simulink model "Modelo_Ceres_RetroROS"  (R2018b)
settings: Solver=VariableStepAuto  StartTime=0.0  StopTime=200  RelTol=1e-3
undefined symbols (not defined in the file): Angular, gainBruit, K_1, K_2, lim, Linear, Tao_1, Tao_2, X, Z
libraries: robotlib x5, simulink x4, realtime_pacer_lib x2
settings Model: Creator=adrir  LastModifiedBy=root
settings DebuggingCC: LibraryContextMissingDiagnostic=none
settings SFSimCC: SimUseLocalCustomCode=off
settings RTWCC: RTWUseLocalCustomCode=off
settings CodeAppCC: StateflowObjectComments=on

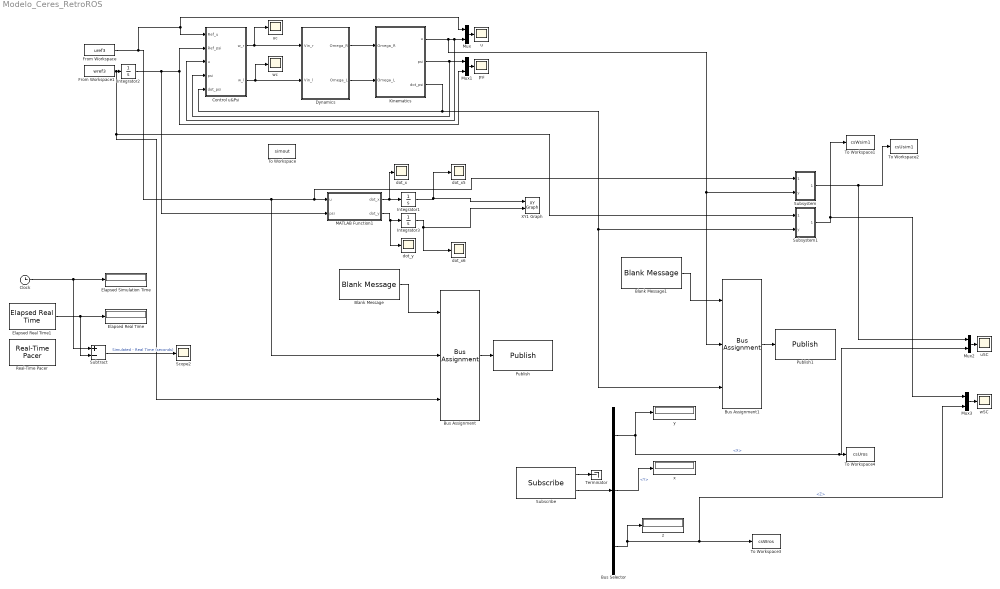
== system Modelo_Ceres_RetroROS ==
  Blank Message : robotlib/Blank Message  messageClass=Message  entityType=geometry_msgs/Twist  messageType=geometry_msgs/Twist  SampleTime=-1
      settings: SourceProductBaseCode=RO
  Blank Message1 : robotlib/Blank Message  messageClass=Message  entityType=geometry_msgs/Vector3  messageType=geometry_msgs/Vector3  SampleTime=-1
      settings: SourceProductBaseCode=RO
  Bus Assignment : BusAssignment  AssignedSignals=Linear.X,Angular.Z
  Bus Assignment1 : BusAssignment  AssignedSignals=X,Z
  Bus Selector : BusSelector  OutputSignals=X,Y,Z
  Clock : Clock
  Control u&Psi : Subsystem
  Dynamics : Subsystem
  Elapsed Real Time : Display
      settings: Decimation=2
  Elapsed Real Time1 : realtime_pacer_lib/Elapsed Real Time
  Elapsed Simulation Time : Display
      settings: Decimation=2
  From Workspace : FromWorkspace  VariableName=uref3
  From Workspace1 : FromWorkspace  VariableName=wref3
  Integrator1 : Integrator
  Integrator2 : Integrator
  Integrator3 : Integrator
  Kinematics : Subsystem
  MATLAB Function1 : MATLAB Function  TreatAsAtomicUnit=on
  Mux{,1..3} (4 alike) : Mux  Inputs=2
  Publish : robotlib/Publish  topicSource=Specify your own  topic=/ceres/cmd_vel  messageType=geometry_msgs/Twist  messageQueueLength=1
      settings: SourceProductBaseCode=RO
  Publish1 : robotlib/Publish  topicSource=Specify your own  topic=/advanced_navigation_driver/twist2D  messageType=geometry_msgs/Vector3  messageQueueLength=1
      settings: SourceProductBaseCode=RO
  Real-Time Pacer : realtime_pacer_lib/Real-Time Pacer  simTimePerRealTime=1
  Scope2 : Scope
  Subscribe : robotlib/Subscribe  topicSource=Select from ROS network  topic=/ceres/controlSignal  messageType=geometry_msgs/Vector3  sampleTime=-1  messageQueueLength=1
      settings: SourceProductBaseCode=RO
  Subsystem : Subsystem
  Subsystem1 : Subsystem
  Subtract : Sum  Inputs=+-
  Terminator : Terminator
  To Workspace : ToWorkspace  VariableName=simout  SaveFormat=Timeseries  SampleTime=-1
  To Workspace1 : ToWorkspace  VariableName=csWsim1  SaveFormat=Timeseries  SampleTime=-1
  To Workspace2 : ToWorkspace  VariableName=csUsim1  SaveFormat=Timeseries  SampleTime=-1
  To Workspace3 : ToWorkspace  VariableName=csWros  SaveFormat=Timeseries  SampleTime=-1
  To Workspace4 : ToWorkspace  VariableName=csUros  SaveFormat=Timeseries  SampleTime=-1
  XY1 Graph : simulink/Sinks/XY Graph  xmin=-30  xmax=30  ymin=-30  ymax=30  st=-1
  dot_x : Scope
  dot_x5 : Scope
  dot_x6 : Scope
  dot_y : Scope
  psi : Scope
  u : Scope
  uSC : Scope
  uc : Scope
  wSC : Scope
  wc : Scope
  x : Display
  y : Display
  z : Display
  wires:
  Dynamics/1(Omega_R) -> Kinematics/1(Omega_R)
  Dynamics/2(Omega_L) -> Kinematics/2(Omega_L)
  Kinematics/2(psi) -> Control u&Psi/4(psi), Mux1/1
  From Workspace/1 -> Control u&Psi/1(Ref_u), Mux/1, Bus Assignment/2, Subsystem/1(Ref), MATLAB Function1/1(u)
  Integrator2/1 -> Control u&Psi/2(Ref_psi), Mux1/2, MATLAB Function1/2(psi)
  Mux/1 -> u/1
  Mux1/1 -> psi/1
  Control u&Psi/1(w_r) -> uc/1, Dynamics/1(Vin_r)
  Control u&Psi/2(w_l) -> wc/1, Dynamics/2(Vin_l)
  Elapsed Real Time1/1 -> Elapsed Real Time/1, Subtract/2
  Subtract/1 -> Scope2/1  "Simulated - Real Time (seconds)"
  Integrator1/1 -> XY1 Graph/1, dot_x5/1
  Bus Assignment/1 -> Publish/1
  From Workspace1/1 -> Subsystem1/1(Ref), Bus Assignment/3, Integrator2/1
  MATLAB Function1/1(dot_x) -> dot_x/1, Integrator1/1
  Integrator3/1 -> XY1 Graph/2, dot_x6/1
  Blank Message/1 -> Bus Assignment/1
  MATLAB Function1/2(dot_y) -> dot_y/1, Integrator3/1
  Clock/1 -> Elapsed Simulation Time/1, Subtract/1
  Kinematics/1(u) -> Bus Assignment1/2, Subsystem/2(y), Control u&Psi/3(u), Mux/2
  Kinematics/3(dot_psi) -> Subsystem1/2(y), Bus Assignment1/3, Control u&Psi/5(dot_psi)
  Bus Assignment1/1 -> Publish1/1
  Blank Message1/1 -> Bus Assignment1/1
  Bus Selector/3 -> z/1, Mux3/2, To Workspace3/1  "<Z>"
  Subscribe/1 -> Terminator/1
  Subscribe/2 -> Bus Selector/1
  Bus Selector/2 -> x/1  "<Y>"
  Bus Selector/1 -> y/1, Mux2/2, To Workspace4/1  "<X>"
  Subsystem/1(c_u) -> Mux2/1, To Workspace2/1
  Subsystem1/1(c_psi) -> Mux3/1, To Workspace1/1
  Mux2/1 -> uSC/1
  Mux3/1 -> wSC/1

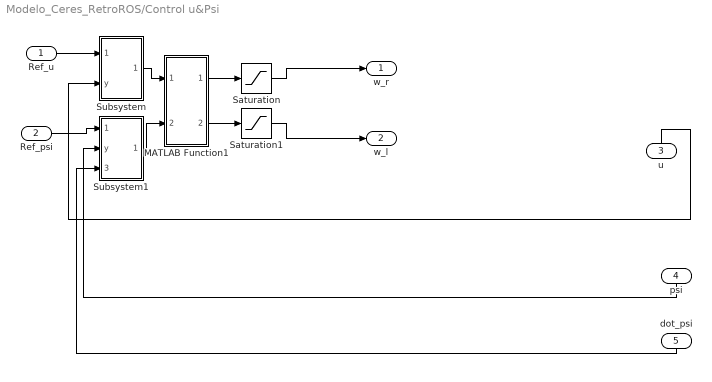
== system Modelo_Ceres_RetroROS/Control u&Psi ==
  Ref_u : Inport
  Ref_psi : Inport  Port=2
  u : Inport  Port=3
  psi : Inport  Port=4
  dot_psi : Inport  Port=5
  MATLAB Function1 : MATLAB Function  TreatAsAtomicUnit=on
  Saturation : Saturate  UpperLimit=10  LowerLimit=-10
  Saturation1 : Saturate  UpperLimit=10  LowerLimit=-10
  Subsystem : Subsystem
  Subsystem1 : Subsystem
  w_r : Outport
  w_l : Outport  Port=2
  wires:
  psi/1 -> Subsystem1/2(y)
  Ref_psi/1 -> Subsystem1/1(Ref)
  Subsystem1/1(c_psi) -> MATLAB Function1/2(c_psi)
  Ref_u/1 -> Subsystem/1(Ref)
  MATLAB Function1/2(w_L) -> Saturation1/1
  Subsystem/1(c_u) -> MATLAB Function1/1(c_u)
  MATLAB Function1/1(w_R) -> Saturation/1
  u/1 -> Subsystem/2(y)
  Saturation/1 -> w_r/1
  Saturation1/1 -> w_l/1
  dot_psi/1 -> Subsystem1/3(dot_y)

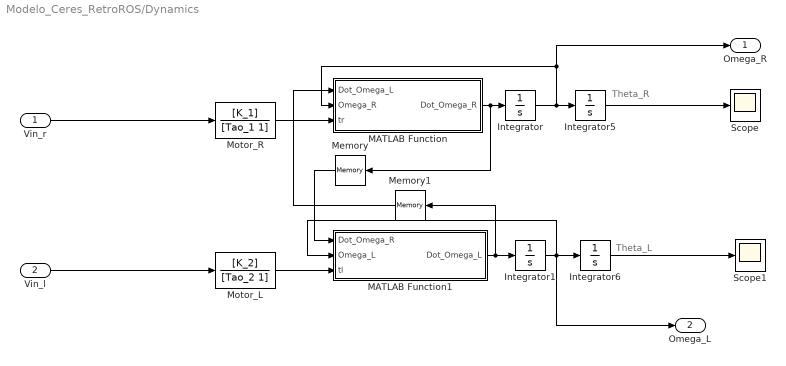
== system Modelo_Ceres_RetroROS/Dynamics ==
  note: Theta_R
  note: Theta_L
  Vin_r : Inport
  Vin_l : Inport  Port=2
  Integrator{,1,5..6} (4 alike) : Integrator
  MATLAB Function : MATLAB Function  TreatAsAtomicUnit=on
  MATLAB Function1 : MATLAB Function  TreatAsAtomicUnit=on
  Memory : Memory
  Memory1 : Memory
  Motor_L : TransferFcn  Numerator=[K_2]  Denominator=[Tao_2 1]
  Motor_R : TransferFcn  Numerator=[K_1]  Denominator=[Tao_1 1]
  Scope : Scope
  Scope1 : Scope
  Omega_R : Outport
  Omega_L : Outport  Port=2
  wires:
  Memory1/1 -> MATLAB Function/1(Dot_Omega_L)
  Memory/1 -> MATLAB Function1/1(Dot_Omega_R)
  Motor_L/1 -> MATLAB Function1/3(tl)
  Integrator5/1 -> Scope/1
  Integrator6/1 -> Scope1/1
  Motor_R/1 -> MATLAB Function/3(tr)
  MATLAB Function1/1(Dot_Omega_L) -> Memory1/1, Integrator1/1
  Integrator/1 -> Integrator5/1, Omega_R/1, MATLAB Function/2(Omega_R)
  MATLAB Function/1(Dot_Omega_R) -> Memory/1, Integrator/1
  Integrator1/1 -> Omega_L/1, MATLAB Function1/2(Omega_L), Integrator6/1
  Vin_l/1 -> Motor_L/1
  Vin_r/1 -> Motor_R/1

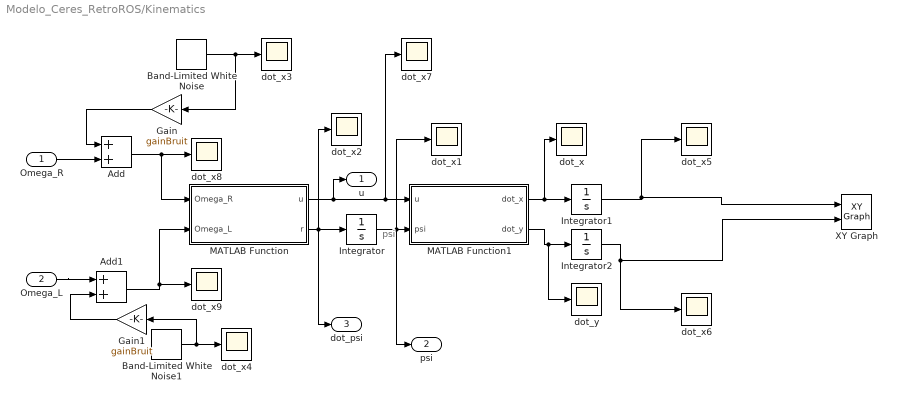
== system Modelo_Ceres_RetroROS/Kinematics ==
  note: psi
  Omega_R : Inport
  Omega_L : Inport  Port=2
  Add : Sum
  Add1 : Sum
  Band-Limited White Noise : simulink/Sources/Band-Limited White Noise  Cov=[0.0005]  Ts=1  seed=[23341]
  Band-Limited White Noise1 : simulink/Sources/Band-Limited White Noise  Cov=[0.0005]  Ts=1  seed=[23341]
  Gain : Gain  Gain=gainBruit
  Gain1 : Gain  Gain=gainBruit
  Integrator : Integrator
  Integrator1 : Integrator
  Integrator2 : Integrator
  MATLAB Function : MATLAB Function  TreatAsAtomicUnit=on
  MATLAB Function1 : MATLAB Function  TreatAsAtomicUnit=on
  XY Graph : simulink/Sinks/XY Graph  xmin=-lim  xmax=lim  ymin=-lim  ymax=lim  st=-1
  dot_x{,1..9} (10 alike) : Scope
  dot_y : Scope
  u : Outport
  psi : Outport  Port=2
  dot_psi : Outport  Port=3
  wires:
  MATLAB Function/2(r) -> dot_psi/1, dot_x2/1, Integrator/1
  MATLAB Function/1(u) -> dot_x7/1, MATLAB Function1/1(u), u/1
  MATLAB Function1/2(dot_y) -> dot_y/1, Integrator2/1
  Integrator2/1 -> XY Graph/2, dot_x6/1
  MATLAB Function1/1(dot_x) -> dot_x/1, Integrator1/1
  Integrator1/1 -> XY Graph/1, dot_x5/1
  Band-Limited White Noise/1 -> Gain/1, dot_x3/1
  Omega_R/1 -> Add/2
  Omega_L/1 -> Add1/1
  Add1/1 -> dot_x9/1, MATLAB Function/2(Omega_L)
  Add/1 -> dot_x8/1, MATLAB Function/1(Omega_R)
  Band-Limited White Noise1/1 -> Gain1/1, dot_x4/1
  Integrator/1 -> MATLAB Function1/2(psi), psi/1, dot_x1/1
  Gain/1 -> Add/1
  Gain1/1 -> Add1/2

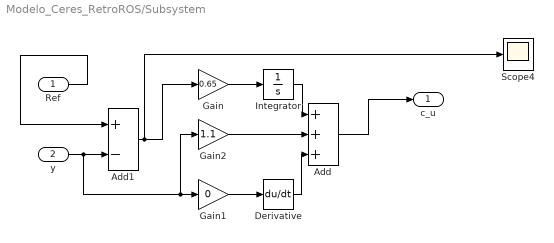
== system Modelo_Ceres_RetroROS/Subsystem ==
  Ref : Inport
  y : Inport  Port=2
  Add : Sum  Inputs=+++
  Add1 : Sum  Inputs=+-
  Derivative : Derivative
  Gain : Gain  Gain=0.65
  Gain1 : Gain  Gain=0
  Gain2 : Gain  Gain=1.1
  Integrator : Integrator
  Scope4 : Scope
  c_u : Outport
  wires:
  Add1/1 -> Scope4/1, Gain/1
  Derivative/1 -> Add/3
  Gain2/1 -> Add/2
  Ref/1 -> Add1/1
  Gain1/1 -> Derivative/1
  Add/1 -> c_u/1
  Gain/1 -> Integrator/1
  y/1 -> Gain2/1, Gain1/1, Add1/2
  Integrator/1 -> Add/1

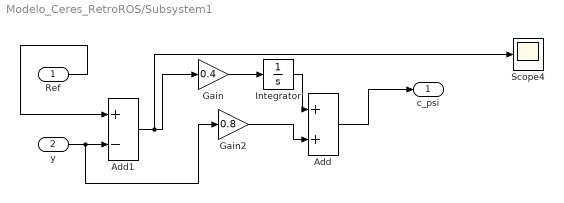
== system Modelo_Ceres_RetroROS/Subsystem1 ==
  Ref : Inport
  y : Inport  Port=2
  Add : Sum
  Add1 : Sum  Inputs=+-
  Gain : Gain  Gain=0.4
  Gain2 : Gain  Gain=0.8
  Integrator : Integrator
  Scope4 : Scope
  c_psi : Outport
  wires:
  Integrator/1 -> Add/1
  y/1 -> Gain2/1, Add1/2
  Gain/1 -> Integrator/1
  Add/1 -> c_psi/1
  Ref/1 -> Add1/1
  Gain2/1 -> Add/2
  Add1/1 -> Scope4/1, Gain/1

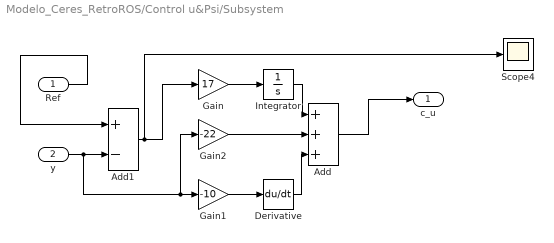
== system Modelo_Ceres_RetroROS/Control u&Psi/Subsystem ==
  Ref : Inport
  y : Inport  Port=2
  Add : Sum  Inputs=+++
  Add1 : Sum  Inputs=+-
  Derivative : Derivative
  Gain : Gain  Gain=17
  Gain1 : Gain  Gain=-10
  Gain2 : Gain  Gain=-22
  Integrator : Integrator
  Scope4 : Scope
  c_u : Outport
  wires:
  Add1/1 -> Scope4/1, Gain/1
  Derivative/1 -> Add/3
  Gain2/1 -> Add/2
  Ref/1 -> Add1/1
  Gain1/1 -> Derivative/1
  Add/1 -> c_u/1
  Gain/1 -> Integrator/1
  y/1 -> Gain2/1, Gain1/1, Add1/2
  Integrator/1 -> Add/1

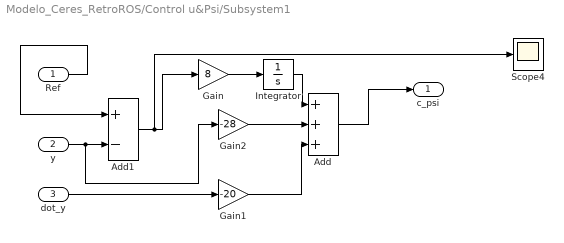
== system Modelo_Ceres_RetroROS/Control u&Psi/Subsystem1 ==
  Ref : Inport
  y : Inport  Port=2
  dot_y : Inport  Port=3
  Add : Sum  Inputs=+++
  Add1 : Sum  Inputs=+-
  Gain : Gain  Gain=8
  Gain1 : Gain  Gain=-20
  Gain2 : Gain  Gain=-28
  Integrator : Integrator
  Scope4 : Scope
  c_psi : Outport
  wires:
  Integrator/1 -> Add/1
  y/1 -> Gain2/1, Add1/2
  Gain/1 -> Integrator/1
  Add/1 -> c_psi/1
  Ref/1 -> Add1/1
  Gain2/1 -> Add/2
  Gain1/1 -> Add/3
  Add1/1 -> Scope4/1, Gain/1
  dot_y/1 -> Gain1/1

== matlab function Modelo_Ceres_RetroROS/Dynamics/MATLAB Function1 ==
  data: Dot_Omega_R input; Omega_L input; tl input; Dot_Omega_L output
function Dot_Omega_L  = fcn(Dot_Omega_R,Omega_L,tl)
b=0.869;	% Center mass to midpoint traction
a=2.255/2;	%distance between front wheels
m=602;		%Total mass
r=0.28;		%Ratio front whell
Iq=588.1;	%Inertia around Z axis
Io=0.0006;	%Inertia motor 
Be=0.02;	%Friction coefficient motor

D11=((m*r*r)/4)+((Iq+m*b*b)*r*r/(4*a*a)+Io);
D22=D11;
D12=(((m*r*r)/4)-((Iq+m*b*b)*r*r/(4*a*a)));
D21=D12;
Beta_3=D11;
Beta_4=D22;



%Dot_Omega_R = (1/D11)*(tr-D12*Dot_Omega_L-Beta_3*Omega_R);
Dot_Omega_L = (1/D11)*(tl-D21*Dot_Omega_R-Beta_4*Omega_L);

== matlab function Modelo_Ceres_RetroROS/Dynamics/MATLAB Function ==
  data: Dot_Omega_L input; Omega_R input; Dot_Omega_R output; tr input
function Dot_Omega_R  = fcn(Dot_Omega_L,Omega_R,tr)
b=0.869;	% Center mass to midpoint traction
a=2.255/2;	%distance between front wheels
m=602;		%Total mass
r=0.28;		%Ratio front whell
Iq=588.1;	%Inertia around Z axis
Io=0.0006;	%Inertia motor 
Be=0.02;	%Friction coefficient motor

D11=((m*r*r)/4)+((Iq+m*b*b)*r*r/(4*a*a)+Io);
D22=D11;
D12=(((m*r*r)/4)-((Iq+m*b*b)*r*r/(4*a*a)));
D21=D12;
Beta_3=D11;
Beta_4=D22;



Dot_Omega_R = (1/D11)*(tr-D12*Dot_Omega_L-Beta_3*Omega_R);
%Dot_Omega_L = (1/D11)*(tl-D21*Dot_Omega_R-Beta_4*Omega_L);

== matlab function Modelo_Ceres_RetroROS/Kinematics/MATLAB Function ==
  data: Omega_R input; Omega_L input; u output; r output
function [u,r]  = fcn(Omega_R,Omega_L)
b=0.869;	% Center mass to midpoint traction
a=2.255/2;	%distance between front wheels
m=602;		%Total mass
r=0.28;		%Ratio front whell
Iq=588.1;	%Inertia around Z axis
Io=0.0006;	%Inertia motor 
Be=0.02;	%Friction coefficient motor


u = (1/2)*(Omega_R+Omega_L);
r = (1/(2*a))*(Omega_R-Omega_L);

== matlab function Modelo_Ceres_RetroROS/Kinematics/MATLAB Function1 ==
  data: u input; psi input; dot_x output; dot_y output
function [dot_x,dot_y]  = fcn(u,psi)
b=0.869;	% Center mass to midpoint traction
a=2.255/2;	%distance between front wheels
m=602;		%Total mass
r=0.28;		%Ratio front whell
Iq=588.1;	%Inertia around Z axis
Io=0.0006;	%Inertia motor 
Be=0.02;	%Friction coefficient motor


dot_x = (u/2)*(cos(psi));
dot_y = (u/2)*(sin(psi));

== matlab function Modelo_Ceres_RetroROS/Control u&Psi/MATLAB Function1 ==
  data: c_u input; c_psi input; w_R output; w_L output
function [w_R,w_L]  = fcn(c_u,c_psi)
b=0.869;	% Center mass to midpoint traction
a=2.255/2;	%distance between front wheels
m=602;		%Total mass
r=0.28;		%Ratio front whell
Iq=588.1;	%Inertia around Z axis
Io=0.0006;	%Inertia motor 
Be=0.02;	%Friction coefficient motor


w_R = (c_u+a*c_psi);
w_L = (c_u-a*c_psi);

== matlab function Modelo_Ceres_RetroROS/MATLAB Function1 ==
  data: u input; psi input; dot_x output; dot_y output
function [dot_x,dot_y]  = fcn(u,psi)
b=0.869;	% Center mass to midpoint traction
a=2.255/2;	%distance between front wheels
m=602;		%Total mass
r=0.28;		%Ratio front whell
Iq=588.1;	%Inertia around Z axis
Io=0.0006;	%Inertia motor 
Be=0.02;	%Friction coefficient motor


dot_x = (u/2)*(cos(psi));
dot_y = (u/2)*(sin(psi));
